simulink model "WS10_03_G10"  (R2019b)
settings: Solver=VariableStepAuto  StartTime=0.0  StopTime=inf  RelTol=1e-3
undefined symbols (not defined in the file): Angular, Linear
libraries: robotlib x12, dspfdesign x1, simulink x1
settings Model: Creator=Azhxt  LastModifiedBy=Azhxt

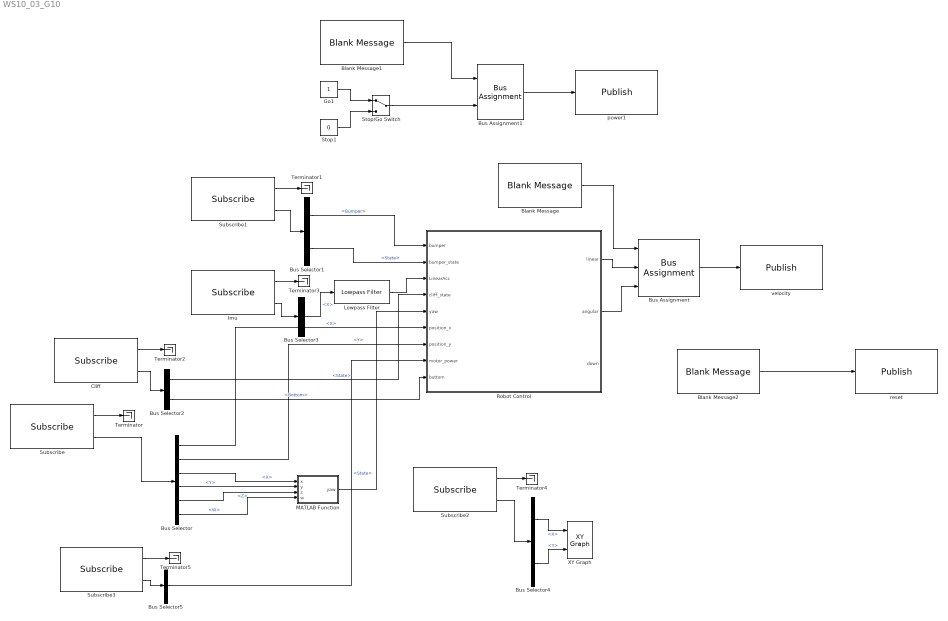
== system WS10_03_G10 ==
  Blank Message : robotlib/Blank Message  messageClass=Message  entityType=geometry_msgs/Twist  messageType=geometry_msgs/Twist  SampleTime=0.01
      settings: SourceProductName=ROS Toolbox
  Blank Message1 : robotlib/Blank Message  messageClass=Message  entityType=kobuki_msgs/MotorPower  messageType=kobuki_msgs/MotorPower  SampleTime=inf
      settings: SourceProductName=ROS Toolbox
  Blank Message2 : robotlib/Blank Message  messageClass=Message  entityType=std_msgs/Empty  messageType=std_msgs/Empty  SampleTime=inf
      settings: SourceProductName=ROS Toolbox
  Bus Assignment : BusAssignment  AssignedSignals=Linear.X,Angular.Z
  Bus Assignment1 : BusAssignment  AssignedSignals=State
  Bus Selector : BusSelector  OutputSignals=Pose.Pose.Position.X,Pose.Pose.Position.Y,Pose.Pose.Orientation.X,Pose.Pose.Orientation.Y,Pose.Pose.Orientation.Z,Pose.Pose.Orientation.W
  Bus Selector1 : BusSelector  OutputSignals=Bumper,State
  Bus Selector2 : BusSelector  OutputSignals=State,Bottom
  Bus Selector3 : BusSelector  OutputSignals=LinearAcceleration.X
  Bus Selector4 : BusSelector  OutputSignals=Pose.Pose.Position.X,Pose.Pose.Position.Y
  Bus Selector5 : BusSelector  OutputSignals=State
  Cliff : robotlib/Subscribe  topicSource=Select from ROS network  topic=/mobile_base/events/cliff  messageType=kobuki_msgs/CliffEvent  sampleTime=-1  messageQueueLength=1
      settings: SourceProductName=ROS Toolbox
  Go1 : Constant  OutDataTypeStr=uint8
  Imu : robotlib/Subscribe  topicSource=Select from ROS network  topic=/mobile_base/sensors/imu_data  messageType=sensor_msgs/Imu  sampleTime=-1  messageQueueLength=1
      settings: SourceProductName=ROS Toolbox
  Lowpass Filter : dspfdesign/Lowpass Filter  FilterType=IIR  DesignForMinimumOrder=on  FilterOrder=50  PassbandFrequency=10  StopbandFrequency=12  PassbandRipple=0.1  StopbandAttenuation=100  InheritSampleRate=off  SampleRate=50  SimulateUsing=Interpreted execution  roundingMode=Floor  coeffsDataTypeStr=fixdt(1,16)
  MATLAB Function : MATLAB Function  TreatAsAtomicUnit=on
  Robot Control : Stateflow chart  BlockKeywords=__PRM__SERIALIZED__DATA__:Stateflow Chart,Stateflow Diagram  TreatAsAtomicUnit=on
  Stop/Go Switch : ManualSwitch
  Stop1 : Constant  Value=0  OutDataTypeStr=uint8
  Subscribe : robotlib/Subscribe  topicSource=Select from ROS network  topic=/odom  messageType=nav_msgs/Odometry  sampleTime=-1  messageQueueLength=1
      settings: SourceProductName=ROS Toolbox
  Subscribe1 : robotlib/Subscribe  topicSource=Select from ROS network  topic=/mobile_base/events/bumper  messageType=kobuki_msgs/BumperEvent  sampleTime=-1  messageQueueLength=1
      settings: SourceProductName=ROS Toolbox
  Subscribe2 : robotlib/Subscribe  topicSource=Select from ROS network  topic=/odom  messageType=nav_msgs/Odometry  sampleTime=-1  messageQueueLength=1
      settings: SourceProductName=ROS Toolbox
  Subscribe3 : robotlib/Subscribe  topicSource=Select from ROS network  topic=/mobile_base/commands/motor_power  messageType=kobuki_msgs/MotorPower  sampleTime=-1  messageQueueLength=1
      settings: SourceProductName=ROS Toolbox
  Terminator{,1..5} (6 alike) : Terminator
  XY Graph : simulink/Sinks/XY Graph  xmin=-5  xmax=5  ymin=-5  ymax=5  st=-1
  power1 : robotlib/Publish  topicSource=Select from ROS network  topic=/mobile_base/commands/motor_power  messageType=kobuki_msgs/MotorPower  messageQueueLength=1
      settings: SourceProductName=ROS Toolbox
  reset : robotlib/Publish  topicSource=Select from ROS network  topic=/mobile_base/commands/reset_odometry  messageType=std_msgs/Empty  messageQueueLength=1
      settings: SourceProductName=ROS Toolbox
  velocity : robotlib/Publish  topicSource=Select from ROS network  topic=/mobile_base/commands/velocity  messageType=geometry_msgs/Twist  messageQueueLength=1
      settings: SourceProductName=ROS Toolbox
  wires:
  Bus Selector1/2 -> Robot Control/2(bumper_state)  "<State>"
  Bus Selector1/1 -> Robot Control/1(bumper)  "<Bumper>"
  Subscribe1/2 -> Bus Selector1/1
  Subscribe1/1 -> Terminator1/1
  Cliff/1 -> Terminator2/1
  Cliff/2 -> Bus Selector2/1
  Imu/2 -> Bus Selector3/1
  Imu/1 -> Terminator3/1
  Stop/Go Switch/1 -> Bus Assignment1/2
  Blank Message1/1 -> Bus Assignment1/1
  Bus Assignment1/1 -> power1/1
  Go1/1 -> Stop/Go Switch/1
  Stop1/1 -> Stop/Go Switch/2
  Robot Control/1(linear) -> Bus Assignment/2
  Robot Control/2(angular) -> Bus Assignment/3
  Bus Assignment/1 -> velocity/1
  Blank Message/1 -> Bus Assignment/1
  Bus Selector2/1 -> Robot Control/4(cliff_state)  "<State>"
  Bus Selector3/1 -> Lowpass Filter/1  "<X>"
  Lowpass Filter/1 -> Robot Control/3(LinearAcc)
  Bus Selector/5 -> MATLAB Function/3(z)  "<Z>"
  Bus Selector/4 -> MATLAB Function/2(y)  "<Y>"
  Bus Selector/3 -> MATLAB Function/1(x)  "<X>"
  Subscribe/1 -> Terminator/1
  Bus Selector/6 -> MATLAB Function/4(w)  "<W>"
  Subscribe/2 -> Bus Selector/1
  MATLAB Function/1(yaw) -> Robot Control/5(yaw)
  Bus Selector/1 -> Robot Control/6(position_x)  "<X>"
  Bus Selector/2 -> Robot Control/7(position_y)  "<Y>"
  Subscribe2/1 -> Terminator4/1
  Subscribe2/2 -> Bus Selector4/1
  Bus Selector4/1 -> XY Graph/1  "<X>"
  Bus Selector4/2 -> XY Graph/2  "<Y>"
  Subscribe3/1 -> Terminator5/1
  Subscribe3/2 -> Bus Selector5/1
  Bus Selector5/1 -> Robot Control/8(motor_power)  "<State>"
  Bus Selector2/2 -> Robot Control/9(buttom)  "<Bottom>"
  Blank Message2/1 -> reset/1

== matlab function WS10_03_G10/MATLAB Function ==
  data: x input; yaw output; y input; z input; w input
function yaw = fcn(x, y, z, w)
%     roll = atan2(2*(w.*x+z.*y),(1-2*(x.^2+y.^2)));
%     pitch = asin(2*(w.*y - z.*x));
    yaw = atan2(2*(w.*z+x.*y),(1-2*(y.^2+z.^2)));
end

== stateflow chart WS10_03_G10/Robot Control ==
  state reverse_cliff
    en:
    current_x = position_x;
    current_y = position_y;
    linear = -0.4;
    angular = 0;
  state down_forward
    en:
    linear = 0.16;
    angular = 0;
  state stop
    en:
    linear = 0
  state cache
  state judge_position
  state reverse_bumper
    en:
    linear = -0.4;
    angular = 0;
    current_x = position_x;
    current_y = position_y;
  state reverse_cliff_onslope
    entry: linear = -0.2;
    entry: angular = 0;
  state position_right
  state initial
    en:
    down = 0;
    yaw_bias = 0;
    first_cliff = 1;
    current_x = position_x;
    current_y = position_y;
  state position_left
  state downslope
  state forwards
    en:
    linear = 0.3;
    angular = 0;
  state turn_right
    entry: angular = -0.7;
    entry: linear = 0;
  state position_record
    en:
    current_x = position_x;
    current_y = position_y;
  state turn_left
    entry: angular = 0.7;
    entry: linear = 0;
  state judge_orientation
  state turn_right1
    en:
    angular=-0.6;
    linear = 0;
  state turn_left1
    en:
    angular=0.6;
    linear = 0;
  state finish_reset_ori
  reverse_cliff -> judge_position : [after(0.2,sec)||((position_x-current_x)^2+(position_y-current_y)^2>0.06)]
  down_forward -> cache [order 1] : [LinearAcc>-0.15]
  forwards -> reverse_cliff [order 2] : [(cliff_state ==1&&buttom<49000)||(cliff_state ==1&&first_cliff ==1)]{linear = 0;first_cliff = 0;}
  cache -> stop [order 1] : [after(0.08,sec)]
  cache -> down_forward [order 2] : [LinearAcc<-0.15]
  down_forward -> reverse_cliff_onslope [order 2] : [cliff_state ==1]{linear = 0;}
  forwards -> down_forward [order 5] : [down == 1]
  reverse_bumper -> judge_position : [after(0.2,sec)||((position_x-current_x)^2+(position_y-current_y)^2>0.06)]
  judge_position -> position_left [order 1] : [position_y>=0]
  judge_position -> position_right [order 2] : [position_y<0]
  forwards -> reverse_bumper [order 1] : [bumper_state == 1&&down==0]
  (default) -> initial
  reverse_cliff_onslope -> judge_orientation : [after(1,sec)||(position_y>-0.02&&position_y<0.02)]
  position_left -> turn_right [order 1] : [yaw>-0.9]
  position_left -> turn_left [order 2] : [yaw<=-0.9]
  position_right -> turn_right [order 2] : [yaw>0.9]
  position_right -> turn_left [order 1] : [yaw<0.9]
  initial -> forwards : [motor_power==1]
  forwards -> downslope [order 4] : [after(0.05,sec)&&LinearAcc<-0.35]
  downslope -> forwards [order 2] : [LinearAcc>-0.35]
  downslope -> judge_orientation [order 1] : [after(0.1,sec)]{down = 1;}
  forwards -> judge_orientation [order 3] : [after(0.6,sec)||((position_x-current_x)^2+(position_y-current_y)^2>0.3)]
  position_record -> forwards
  turn_right -> position_record : [(after(0.5,sec)&&(yaw<yaw_bias+0.45))||yaw<-1.4+yaw_bias]
  turn_left -> position_record : [(after(0.5,sec)&&yaw>yaw_bias-0.45)||yaw>1.4+yaw_bias]
  finish_reset_ori -> position_record
  judge_orientation -> turn_right1 [order 1] : [yaw>=yaw_bias]
  judge_orientation -> turn_left1 [order 2] : [yaw<yaw_bias]
  turn_left1 -> finish_reset_ori : [yaw>-0.03+yaw_bias&&yaw<yaw_bias+0.03]
  turn_right1 -> finish_reset_ori : [(yaw>-0.05+yaw_bias&&yaw<yaw_bias+0.05)||yaw<-1.5||yaw>1.5]
  data: linear output double =0; bumper input uint8; angular output double; bumper_state input uint8; LinearAcc input; cliff_state input uint8; yaw input; position_x input; yaw_ini local; yaw_nota local; position_y input; x_ini local; y_ini local; yaw_bias local; down output uint8; motor_power input; first_cliff local uint8; buttom input; current_x local; current_y local
